simulink model "ID_model"  (R2015b)
settings: Solver=ode5  StartTime=0.0  StopTime=inf  FixedStep=0.02  RelTol=1e-3
undefined symbols (not defined in the file or in its folder): Angular, Ki_L, Ki_W, Kp_L, Kp_W, Linear, X, Y, Z
libraries: robotlib x18, simulink x2, realtime_pacer_lib x1
settings Model: Creator=root  LastModifiedBy=root

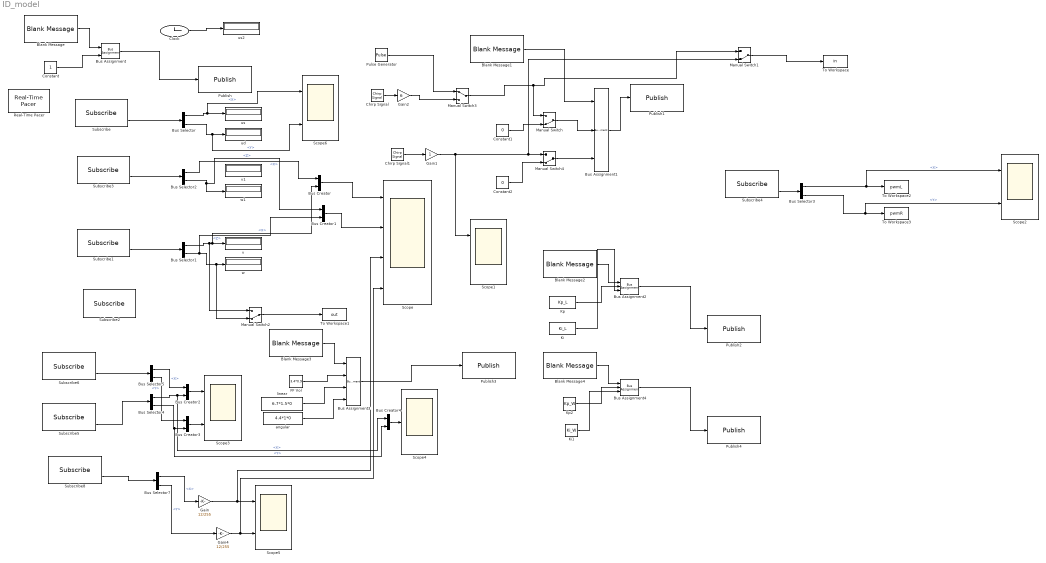
== system ID_model ==
  Blank Message : robotlib/Blank Message  SourceLibraryInfo=This block requires Robotics System Toolbox  messageType=std_msgs/UInt8  SampleTime=inf
  Blank Message1 : robotlib/Blank Message  SourceLibraryInfo=This block requires Robotics System Toolbox  messageType=geometry_msgs/Twist  SampleTime=inf
  Blank Message2 : robotlib/Blank Message  SourceLibraryInfo=This block requires Robotics System Toolbox  messageType=geometry_msgs/Vector3  SampleTime=inf
  Blank Message3 : robotlib/Blank Message  SourceLibraryInfo=This block requires Robotics System Toolbox  messageType=geometry_msgs/Vector3  SampleTime=inf
  Blank Message4 : robotlib/Blank Message  SourceLibraryInfo=This block requires Robotics System Toolbox  messageType=geometry_msgs/Vector3  SampleTime=inf
  Bus Assignment : BusAssignment  AssignedSignals=Data
  Bus Assignment1 : BusAssignment  AssignedSignals=Linear.X,Angular.Z
  Bus Assignment2 : BusAssignment  AssignedSignals=X,Y
  Bus Assignment3 : BusAssignment  AssignedSignals=X,Y,Z
  Bus Assignment4 : BusAssignment  AssignedSignals=X,Y
  Bus Creator{,1..4} (5 alike) : BusCreator  Inputs=2
  Bus Selector{,3..5,7} (5 alike) : BusSelector  OutputSignals=X,Y
  Bus Selector1 : BusSelector  OutputSignals=Linear.X,Angular.Z
  Bus Selector2 : BusSelector  OutputSignals=X,Z
  Chirp Signal : simulink/Sources/Chirp Signal  f1=0.001  T=60  f2=1
  Chirp Signal1 : simulink/Sources/Chirp Signal  f1=0.001  T=60  f2=1
  Clock : Clock
  Constant : Constant  OutDataTypeStr=Inherit: Inherit via back propagation
  Constant1 : Constant  Value=0
  Constant2 : Constant  Value=0
  FF Vol : Constant  Value=3.4*0.9  OutDataTypeStr=Inherit: Inherit via back propagation
  Gain : Gain  Gain=12/255
  Gain1 : Gain
  Gain2 : Gain  Gain=6
  Gain4 : Gain  Gain=12/255
  Ki : Constant  Value=Ki_L  OutDataTypeStr=Inherit: Inherit via back propagation
  Ki1 : Constant  Value=Ki_W  OutDataTypeStr=Inherit: Inherit via back propagation
  Kp : Constant  Value=Kp_L  OutDataTypeStr=Inherit: Inherit via back propagation
  Kp2 : Constant  Value=Kp_W  OutDataTypeStr=Inherit: Inherit via back propagation
  Manual Switch{,1..2,4} (4 alike) : ManualSwitch  CurrentSetting=0
  Manual Switch3 : ManualSwitch
  Publish : robotlib/Publish  SourceLibraryInfo=This block requires Robotics System Toolbox  topicSource=Select from ROS network  topic=/andbot/OpenLoop_Switch  messageType=std_msgs/UInt8  messageQueueLength=1
  Publish1 : robotlib/Publish  SourceLibraryInfo=This block requires Robotics System Toolbox  topicSource=Select from ROS network  topic=/andbot/cmd_vel  messageType=geometry_msgs/Twist  messageQueueLength=1
  Publish2 : robotlib/Publish  SourceLibraryInfo=This block requires Robotics System Toolbox  topicSource=Select from ROS network  topic=/andbot/gain_L  messageType=geometry_msgs/Vector3  messageQueueLength=1
  Publish3 : robotlib/Publish  SourceLibraryInfo=This block requires Robotics System Toolbox  topicSource=Select from ROS network  topic=/andbot/FeedForward_Vol  messageType=geometry_msgs/Vector3  messageQueueLength=1
  Publish4 : robotlib/Publish  SourceLibraryInfo=This block requires Robotics System Toolbox  topicSource=Select from ROS network  topic=/andbot/gain_W  messageType=geometry_msgs/Vector3  messageQueueLength=1
  Pulse Generator : DiscretePulseGenerator  PulseType=Time based  Amplitude=0.5  PulseWidth=50
  Real-Time Pacer : realtime_pacer_lib/Real-Time Pacer  simTimePerRealTime=inf
  Scope : Scope  NumInputPorts=4
  Scope{1..3,5..6} (5 alike) : Scope  NumInputPorts=2
  Scope4 : Scope
  Subscribe : robotlib/Subscribe  SourceLibraryInfo=This block requires Robotics System Toolbox  topicSource=Select from ROS network  topic=/andbot/cmd_us_ud  messageType=geometry_msgs/Vector3  sampleTime=-1  messageQueueLength=1
  Subscribe1 : robotlib/Subscribe  SourceLibraryInfo=This block requires Robotics System Toolbox  topicSource=Select from ROS network  topic=/andbot/feedback_vel  messageType=geometry_msgs/Twist  sampleTime=-1  messageQueueLength=1
  Subscribe2 : robotlib/Subscribe  SourceLibraryInfo=This block requires Robotics System Toolbox  topicSource=Select from ROS network  topic=/andbot/feedback_vel  messageType=geometry_msgs/Twist  sampleTime=-1  messageQueueLength=1
  Subscribe3 : robotlib/Subscribe  SourceLibraryInfo=This block requires Robotics System Toolbox  topicSource=Select from ROS network  topic=/andbot/cmd_vel_mobile_mega  messageType=geometry_msgs/Vector3  sampleTime=-1  messageQueueLength=1
  Subscribe4 : robotlib/Subscribe  SourceLibraryInfo=This block requires Robotics System Toolbox  topicSource=Select from ROS network  topic=/andbot/cmd_wheel_PWM  messageType=geometry_msgs/Vector3  sampleTime=-1  messageQueueLength=1
  Subscribe5 : robotlib/Subscribe  SourceLibraryInfo=This block requires Robotics System Toolbox  topicSource=Select from ROS network  topic=/andbot/feedback_wheel_angularVel  messageType=geometry_msgs/Vector3  sampleTime=-1  messageQueueLength=1
  Subscribe6 : robotlib/Subscribe  SourceLibraryInfo=This block requires Robotics System Toolbox  topicSource=Select from ROS network  topic=/andbot/cmd_wheel_angularVel  messageType=geometry_msgs/Vector3  sampleTime=-1  messageQueueLength=1
  Subscribe8 : robotlib/Subscribe  SourceLibraryInfo=This block requires Robotics System Toolbox  topicSource=Select from ROS network  topic=/andbot/cmd_wheel_PWM  messageType=geometry_msgs/Vector3  sampleTime=-1  messageQueueLength=1
  To Workspace : ToWorkspace  VariableName=in  SaveFormat=Timeseries  SampleTime=-1
  To Workspace1 : ToWorkspace  VariableName=out  SaveFormat=Timeseries  SampleTime=-1
  To Workspace2 : ToWorkspace  VariableName=pwmL  SaveFormat=Timeseries  SampleTime=-1
  To Workspace3 : ToWorkspace  VariableName=pwmR  SaveFormat=Timeseries  SampleTime=-1
  "angular " : Constant  Value=4.4*1*0  OutDataTypeStr=Inherit: Inherit via back propagation
  linear : Constant  Value=6.7*1.5*0  OutDataTypeStr=Inherit: Inherit via back propagation
  ud : Display
  us : Display
  us2 : Display
  v : Display
  v1 : Display
  w : Display
  w1 : Display
  wires:
  Subscribe/2 -> Bus Selector/1
  Bus Selector/1 -> Scope6/1, us/1  "<X>"
  Bus Selector/2 -> Scope6/2, ud/1  "<Y>"
  Subscribe1/2 -> Bus Selector1/1
  Bus Selector1/1 -> Manual Switch2/1, Bus Creator/2, v/1  "<X>"
  Bus Selector1/2 -> Bus Creator1/2, Manual Switch2/2, w/1  "<Z>"
  Bus Creator/1 -> Scope/1
  Subscribe3/2 -> Bus Selector2/1
  Bus Selector2/2 -> Bus Creator1/1, w1/1  "<Z>"
  Bus Selector2/1 -> Bus Creator/1  "<X>"
  Bus Creator1/1 -> Scope/2
  Constant1/1 -> Manual Switch/2
  Manual Switch3/1 -> Manual Switch1/1, Manual Switch/1
  Constant/1 -> Bus Assignment/2
  Blank Message/1 -> Bus Assignment/1
  Bus Assignment/1 -> Publish/1
  Bus Assignment1/1 -> Publish1/1
  Manual Switch/1 -> Bus Assignment1/2
  Blank Message1/1 -> Bus Assignment1/1
  Clock/1 -> us2/1
  Manual Switch1/1 -> To Workspace/1
  Manual Switch2/1 -> To Workspace1/1
  Kp/1 -> Bus Assignment2/2
  Blank Message2/1 -> Bus Assignment2/1
  Bus Assignment2/1 -> Publish2/1
  Ki/1 -> Bus Assignment2/3
  Chirp Signal/1 -> Gain2/1
  FF Vol/1 -> Bus Assignment3/2
  Blank Message3/1 -> Bus Assignment3/1
  Bus Assignment3/1 -> Publish3/1
  Manual Switch4/1 -> Bus Assignment1/3
  Constant2/1 -> Manual Switch4/2
  Chirp Signal1/1 -> Gain1/1
  Kp2/1 -> Bus Assignment4/2
  Blank Message4/1 -> Bus Assignment4/1
  Bus Assignment4/1 -> Publish4/1
  Ki1/1 -> Bus Assignment4/3
  Gain1/1 -> Scope1/1, Manual Switch1/2, Manual Switch4/1
  Gain2/1 -> Manual Switch3/2
  Subscribe4/2 -> Bus Selector3/1
  Bus Selector3/1 -> Scope2/1, To Workspace2/1  "<X>"
  Bus Selector3/2 -> Scope2/2, To Workspace3/1  "<Y>"
  Pulse Generator/1 -> Manual Switch3/1
  Subscribe5/2 -> Bus Selector4/1
  Subscribe6/2 -> Bus Selector5/1
  Bus Creator3/1 -> Scope3/2
  Bus Creator2/1 -> Scope3/1
  Bus Selector5/1 -> Bus Creator2/1  "<X>"
  Bus Selector4/1 -> Bus Creator4/1, Bus Creator2/2  "<X>"
  Bus Selector5/2 -> Bus Creator3/1  "<Y>"
  Bus Selector4/2 -> Bus Creator4/2, Bus Creator3/2  "<Y>"
  Bus Creator4/1 -> Scope4/1
  linear/1 -> Bus Assignment3/3
  "angular "/1 -> Bus Assignment3/4
  Subscribe8/2 -> Bus Selector7/1
  Bus Selector7/1 -> Gain/1  "<X>"
  Bus Selector7/2 -> Gain4/1  "<Y>"
  Gain/1 -> Scope/3, Scope5/1
  Gain4/1 -> Scope/4, Scope5/2
